simulink model "Two_Channel_Telerobotic"  (R2022a)
settings: Solver=ode4  StartTime=0.0  StopTime=60  FixedStep=0.001  MaxStep=0.01
libraries: slpidlib x2
settings Model: Creator=smrit  LastModifiedBy=adhit
settings SolverCC: NumberNewtonIterations=1000  AlgebraicLoopSolver=TrustRegion  AutoInsertRateTranBlk=on  ODENIntegrationMethod=ode8
settings DebuggingCC: UnconnectedInputMsg=warning  UnconnectedOutputMsg=warning  UnconnectedLineMsg=warning  SFMachineParentedDataDiag=warning

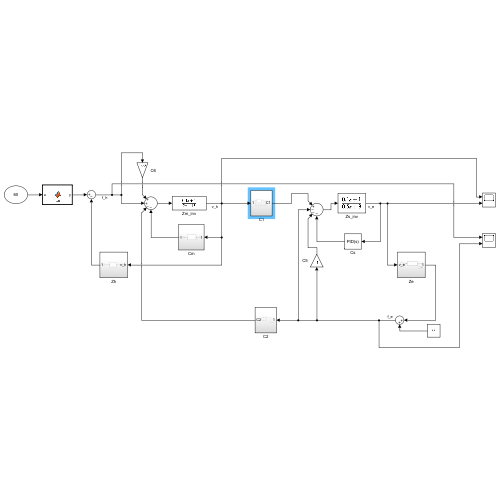
[thumbnail: Simulink's stored preview of the top-level diagram]
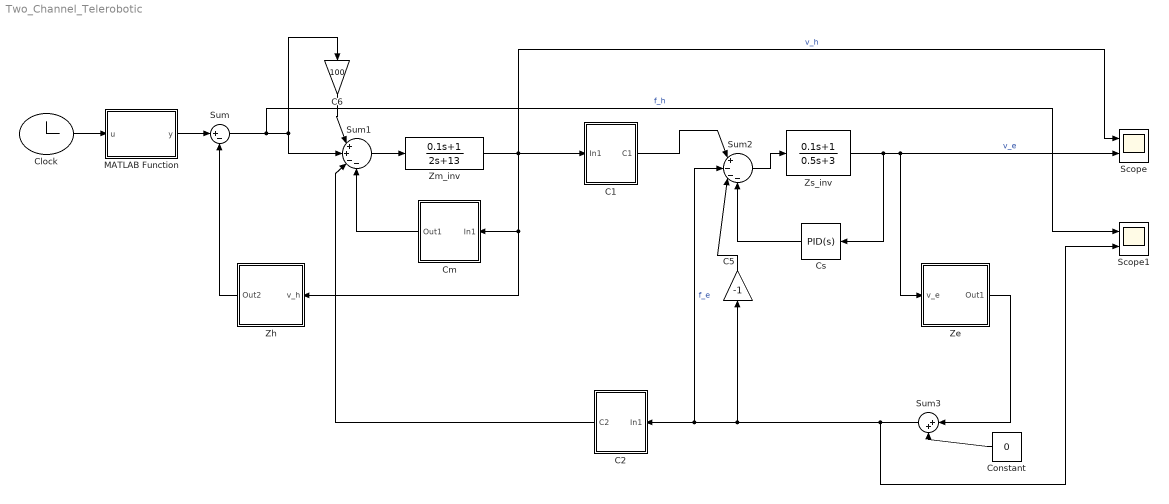
== system Two_Channel_Telerobotic ==
  C1 : Subsystem
  C2 : Subsystem
  C5 : Gain  Gain=-1
  C6 : Gain  Gain=100
  Clock : Clock
  Cm : Subsystem
  Constant : Constant  Value=0
  Cs : slpidlib/PID Controller  Controller=PID  Form=Parallel  TimeDomain=Continuous-time  UseExternalTs=off  SampleTime=-1  IntegratorMethod=Forward Euler  FilterMethod=Forward Euler  ControllerParametersSource=internal  P=100  I=0  UseKiTs=off  D=1  N=1000  UseFilter=on  TunerSelectOption=Transfer Function Based (PID Tuner App)  InitialConditionSource=internal  InitialConditionForIntegrator=0  InitialConditionForFilter=0  DifferentiatorICPrevScaledInput=0  ExternalReset=none  TrackingMode=off  Kt=1  LimitOutput=off  SatLimitsSource=internal  UpperSaturationLimit=inf  LowerSaturationLimit=-inf  LinearizeAsGain=on  AntiWindupMode=none  Kb=1  POutMin=[]  POutMax=[]  IOutMin=[]  IOutMax=[]  DOutMin=[]  DOutMax=[]  NOutMin=[]  NOutMax=[]  SumOutMin=[]  SumOutMax=[]  SaturationOutMin=[]  SaturationOutMax=[]  PParamMin=[]  PParamMax=[]  IParamMin=[]  IParamMax=[]  DParamMin=[]  DParamMax=[]  NParamMin=[]  NParamMax=[]  KbParamMin=[]  KbParamMax=[]  KtParamMin=[]  KtParamMax=[]  KbOutMin=[]  KbOutMax=[]  KtOutMin=[]  KtOutMax=[]  IntegratorOutMin=[]  IntegratorOutMax=[]  FilterOutMin=[]  FilterOutMax=[]  SumI1OutMin=[]  SumI1OutMax=[]  SumI2OutMin=[]  SumI2OutMax=[]  SumI3OutMin=[]  SumI3OutMax=[]  SumI4OutMin=[]  SumI4OutMax=[]  SumDOutMin=[]  SumDOutMax=[]  DifferentiatorOutMin=[]  DifferentiatorOutMax=[]  FilterDiffOutCoefMin=[]  FilterDiffOutCoefMax=[]  ReciprocalOutMin=[]  ReciprocalOutMax=[]  SumDenOutMin=[]  SumDenOutMax=[]  SumNumOutMin=[]  SumNumOutMax=[]  DivideOutMin=[]  DivideOutMax=[]  UdiffTsProdOutMin=[]  UdiffTsProdOutMax=[]  NTsProdOutMin=[]  NTsProdOutMax=[]  UintegralTsProdOutMin=[]  UintegralTsProdOutMax=[]  UngainTsProdOutMin=[]  UngainTsProdOutMax=[]  IntegratorContinuousStateAttributes=''  IntegratorStateMustResolveToSignalObject=off  IntegratorRTWStateStorageClass=Auto  FilterContinuousStateAttributes=''  FilterStateMustResolveToSignalObject=off  FilterRTWStateStorageClass=Auto  ParallelPVariant=InternalParameters  IdealPVariant=Disabled  IVariant=InternalParameters  DVariant=InternalParameters  IntegratorVariant=Continuous  SatVariant=Disabled  AWVariant=Passthrough  PCopyVariant=Disabled  TRVariant=Disabled  FdbkBlocksVariant=Forward  IdealPFdbkVariant=Disabled  SatFdbkVariant=Disabled  DerivativeFilterVariant=ContFilter  NVariant=InternalParameters  NCopyVariant=Disabled  FilterICVariant=InternalICsFilter  IntegratorICVariant=InternalICs  ExternalResetVariant=Disabled  TRSumVariant=Passthrough  SumFdbkVariant=Disabled  SumVariant=Sum_PID  TsampFilterVariant=InternalTs  TsampNgainVariant=Passthrough  TsampIntegralVariant=Passthrough  ExternalSaturationOutDataTypeStr=Inherit: Same as second input  aMode=0
  MATLAB Function : MATLAB Function  TreatAsAtomicUnit=on
  Scope : Scope  NumInputPorts=2
  Scope1 : Scope  NumInputPorts=2
  Sum : Sum  Inputs=|+-
  Sum1 : Sum  Inputs=|++--
  Sum2 : Sum  Inputs=|+---
  Sum3 : Sum  Inputs=|++
  Ze : Subsystem
  Zh : Subsystem
  Zm_inv : TransferFcn  Numerator=[0.1 1]  Denominator=[2 13]  AbsoluteTolerance=0.01
  Zs_inv : TransferFcn  Numerator=[0.1 1]  Denominator=[0.5 3]
  wires:
  C2/1(C2) -> Sum1/3
  Zh/1(Out2) -> Sum/2
  Constant/1 -> Sum3/2
  Zm_inv/1 -> C1/1(In1), Scope/1, Cm/1(In1), Zh/1(v_h)  "v_h"
  Clock/1 -> MATLAB Function/1(u)
  Sum2/1 -> Zs_inv/1
  Sum3/1 -> Scope1/2, C2/1(In1), Sum2/2, C5/1  "f_e"
  Cs/1 -> Sum2/4
  Zs_inv/1 -> Scope/2, Ze/1(v_e), Cs/1  "v_e"
  Sum1/1 -> Zm_inv/1
  Ze/1(Out1) -> Sum3/1
  Sum/1 -> Scope1/1, C6/1, Sum1/2  "f_h"
  C6/1 -> Sum1/1
  C5/1 -> Sum2/3
  C1/1(C1) -> Sum2/1
  MATLAB Function/1(y) -> Sum/1
  Cm/1(Out1) -> Sum1/4

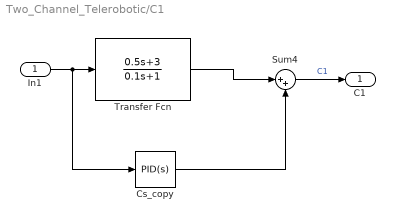
== system Two_Channel_Telerobotic/C1 ==
  In1 : Inport
  Cs_copy : slpidlib/PID Controller  Controller=PID  Form=Parallel  TimeDomain=Continuous-time  UseExternalTs=off  SampleTime=-1  IntegratorMethod=Forward Euler  FilterMethod=Forward Euler  ControllerParametersSource=internal  P=100  I=0  UseKiTs=off  D=1  N=1000  UseFilter=on  TunerSelectOption=Transfer Function Based (PID Tuner App)  InitialConditionSource=internal  InitialConditionForIntegrator=0  InitialConditionForFilter=0  DifferentiatorICPrevScaledInput=0  ExternalReset=none  TrackingMode=off  Kt=1  LimitOutput=off  SatLimitsSource=internal  UpperSaturationLimit=inf  LowerSaturationLimit=-inf  LinearizeAsGain=on  AntiWindupMode=none  Kb=1  POutMin=[]  POutMax=[]  IOutMin=[]  IOutMax=[]  DOutMin=[]  DOutMax=[]  NOutMin=[]  NOutMax=[]  SumOutMin=[]  SumOutMax=[]  SaturationOutMin=[]  SaturationOutMax=[]  PParamMin=[]  PParamMax=[]  IParamMin=[]  IParamMax=[]  DParamMin=[]  DParamMax=[]  NParamMin=[]  NParamMax=[]  KbParamMin=[]  KbParamMax=[]  KtParamMin=[]  KtParamMax=[]  KbOutMin=[]  KbOutMax=[]  KtOutMin=[]  KtOutMax=[]  IntegratorOutMin=[]  IntegratorOutMax=[]  FilterOutMin=[]  FilterOutMax=[]  SumI1OutMin=[]  SumI1OutMax=[]  SumI2OutMin=[]  SumI2OutMax=[]  SumI3OutMin=[]  SumI3OutMax=[]  SumI4OutMin=[]  SumI4OutMax=[]  SumDOutMin=[]  SumDOutMax=[]  DifferentiatorOutMin=[]  DifferentiatorOutMax=[]  FilterDiffOutCoefMin=[]  FilterDiffOutCoefMax=[]  ReciprocalOutMin=[]  ReciprocalOutMax=[]  SumDenOutMin=[]  SumDenOutMax=[]  SumNumOutMin=[]  SumNumOutMax=[]  DivideOutMin=[]  DivideOutMax=[]  UdiffTsProdOutMin=[]  UdiffTsProdOutMax=[]  NTsProdOutMin=[]  NTsProdOutMax=[]  UintegralTsProdOutMin=[]  UintegralTsProdOutMax=[]  UngainTsProdOutMin=[]  UngainTsProdOutMax=[]  IntegratorContinuousStateAttributes=''  IntegratorStateMustResolveToSignalObject=off  IntegratorRTWStateStorageClass=Auto  FilterContinuousStateAttributes=''  FilterStateMustResolveToSignalObject=off  FilterRTWStateStorageClass=Auto  ParallelPVariant=InternalParameters  IdealPVariant=Disabled  IVariant=InternalParameters  DVariant=InternalParameters  IntegratorVariant=Continuous  SatVariant=Disabled  AWVariant=Passthrough  PCopyVariant=Disabled  TRVariant=Disabled  FdbkBlocksVariant=Forward  IdealPFdbkVariant=Disabled  SatFdbkVariant=Disabled  DerivativeFilterVariant=ContFilter  NVariant=InternalParameters  NCopyVariant=Disabled  FilterICVariant=InternalICsFilter  IntegratorICVariant=InternalICs  ExternalResetVariant=Disabled  TRSumVariant=Passthrough  SumFdbkVariant=Disabled  SumVariant=Sum_PID  TsampFilterVariant=InternalTs  TsampNgainVariant=Passthrough  TsampIntegralVariant=Passthrough  ExternalSaturationOutDataTypeStr=Inherit: Same as second input  aMode=0
  Sum4 : Sum  Inputs=|++
  Transfer Fcn : TransferFcn  Numerator=[0.5 3]  Denominator=[0.1 1]
  C1 : Outport
  wires:
  In1/1 -> Transfer Fcn/1, Cs_copy/1
  Cs_copy/1 -> Sum4/2
  Transfer Fcn/1 -> Sum4/1
  Sum4/1 -> C1/1  "C1"

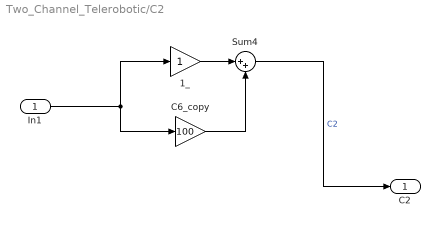
== system Two_Channel_Telerobotic/C2 ==
  In1 : Inport
  1_ : Gain
  C6_copy : Gain  Gain=100
  Sum4 : Sum  Inputs=|++
  C2 : Outport
  wires:
  1_/1 -> Sum4/1
  C6_copy/1 -> Sum4/2
  Sum4/1 -> C2/1  "C2"
  In1/1 -> C6_copy/1, 1_/1

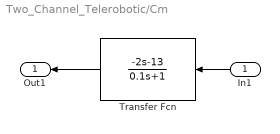
== system Two_Channel_Telerobotic/Cm ==
  In1 : Inport
  Transfer Fcn : TransferFcn  Numerator=[-2 -13]  Denominator=[0.1 1]
  Out1 : Outport
  wires:
  In1/1 -> Transfer Fcn/1
  Transfer Fcn/1 -> Out1/1

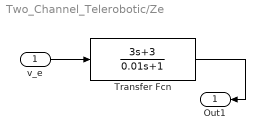
== system Two_Channel_Telerobotic/Ze ==
  v_e : Inport
  Transfer Fcn : TransferFcn  Numerator=[3 3]  Denominator=[0.01 1]
  Out1 : Outport
  wires:
  v_e/1 -> Transfer Fcn/1
  Transfer Fcn/1 -> Out1/1

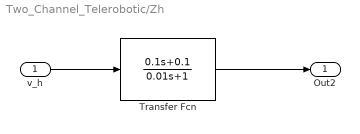
== system Two_Channel_Telerobotic/Zh ==
  v_h : Inport
  Transfer Fcn : TransferFcn  Numerator=[0.1 0.1]  Denominator=[0.01 1]
  Out2 : Outport
  wires:
  v_h/1 -> Transfer Fcn/1
  Transfer Fcn/1 -> Out2/1

== matlab function Two_Channel_Telerobotic/MATLAB Function ==
  data: u input; y output
function y = fcn(u)

y = 20*sin(u)+20*cos(2*u)+20*sin(10*u);
